simulink model "derivative_test"  (R2022b)
settings: Solver=FixedStepDiscrete  StartTime=0.0  StopTime=60  FixedStep=0.001  RelTol=1e-3
libraries: eeGeneralControl x2
settings Model: Creator=doann  LastModifiedBy=doann
settings OptimizationCC: DefaultParameterBehavior=Inlined  UseDivisionForNetSlopeComputation=on  GainParamInheritBuiltInType=on  UseFloatMulNetSlope=on  InlineInvariantSignals=on  PassReuseOutputArgsAs=Individual arguments  ZeroExternalMemoryAtStartup=off  ZeroInternalMemoryAtStartup=off  NoFixptDivByZeroProtection=on  EfficientFloat2IntCast=on  LifeSpan=1  OptimizeBlockOrder=speed  DifferentSizesBufferReuse=on  EfficientTunableParamExpr=on
settings DebuggingCC: ParameterTunabilityLossMsg=error
settings HardwareCC: ProdBitPerPointer=32  ProdBitPerSizeT=32  ProdBitPerPtrDiffT=32  ProdLargestAtomicInteger=Long  ProdLargestAtomicFloat=Double  ProdWordSize=32  ProdLongLongMode=on  ProdHWDeviceType=ARM Compatible->ARM Cortex-M
settings SFSimCC: MATLABDynamicMemAlloc=off
settings RTWCC: Description=Embedded Coder  SystemTargetFile=ert.tlc  GenCodeOnly=on  TemplateMakefile=ert_default_tmf  TargetLang=C++
settings CodeAppCC: ForceParamTrailComments=on  IgnoreCustomStorageClasses=off  OperatorAnnotations=on  SimulinkDataObjDesc=on  SFDataObjDesc=on  CustomSymbolStrGlobalVar=rt$N$M  CustomSymbolStrType=$N$M  CustomSymbolStrFcn=$N$M$F  CustomSymbolStrMacro=$N$M  InsertBlockDesc=on
settings ERTTargetCC: TargetLangStandard=C++11 (ISO)  GenerateSampleERTMain=on  IncludeMdlTerminateFcn=off  CombineSignalStateStructs=on  SuppressErrorStatus=on  SupportAbsoluteTime=off  CodeInterfacePackaging=C++ class  SupportComplex=off  InlinedParameterPlacement=NonHierarchical  RootIOFormat=Structure reference  ERTCustomFileTemplate=example_file_process.tlc  ERTFilePackagingFormat=CompactWithDataFile

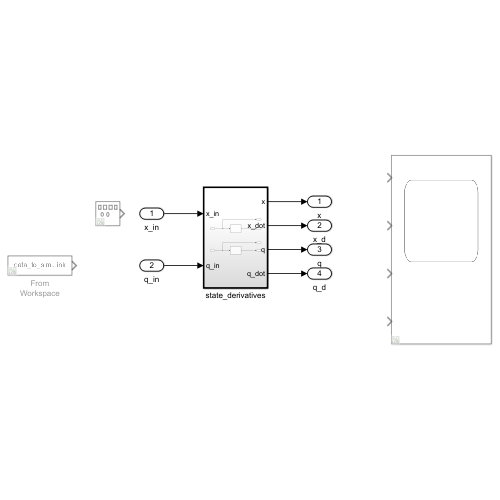
[thumbnail: Simulink's stored preview of the top-level diagram]
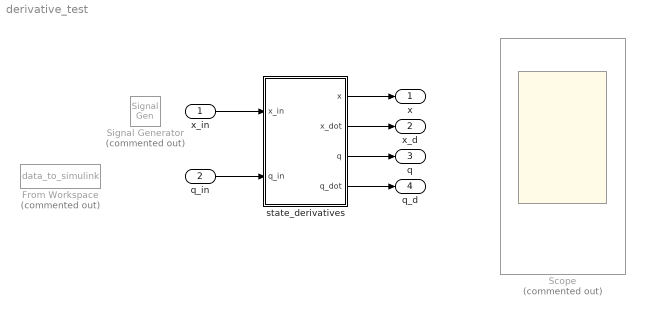
== system derivative_test ==
  x_in : Inport
  q_in : Inport  Port=2
  From Workspace : FromWorkspace  Commented=on  VariableName=data_to_simulink  SampleTime=0.001  OutputAfterFinalValue=Holding final value
  Scope : Scope  Commented=on  NumInputPorts=4
  Signal Generator : SignalGenerator  Commented=on  Amplitude=0.9  Frequency=pi  Units=rad/sec
  state_derivatives : Subsystem  TreatAsAtomicUnit=on  SystemSampleTime=0.001
  x : Outport
  x_d : Outport  Port=2
  q : Outport  Port=3
  q_d : Outport  Port=4
  wires:
  x_in/1 -> state_derivatives/1(x_in)
  q_in/1 -> state_derivatives/2(q_in)
  state_derivatives/1(x) -> x/1
  state_derivatives/2(x_dot) -> x_d/1
  state_derivatives/3(q) -> q/1
  state_derivatives/4(q_dot) -> q_d/1

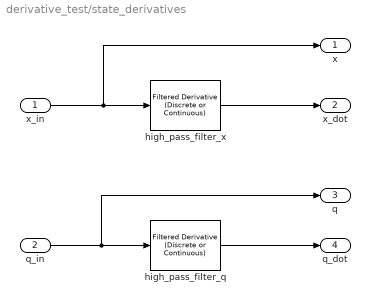
== system derivative_test/state_derivatives ==
  x_in : Inport
  q_in : Inport  Port=2
  high_pass_filter_q : eeGeneralControl/Filtered Derivative (Discrete or Continuous)  K=1  T=0.02  B=inf  A=-inf  minRatio=10  init_option=Inherited from block input  x0=0  Ts=0.001
      settings: LibrarySourceBlock=|
      | ee_sl_lib/General Control/Filtered Derivative
      | (Discrete or Continuous)
  high_pass_filter_x : eeGeneralControl/Filtered Derivative (Discrete or Continuous)  K=1  T=0.02  B=inf  A=-inf  minRatio=10  init_option=Inherited from block input  x0=0  Ts=0.001
      settings: LibrarySourceBlock=|
      | ee_sl_lib/General Control/Filtered Derivative
      | (Discrete or Continuous)
  x : Outport
  x_dot : Outport  Port=2
  q : Outport  Port=3
  q_dot : Outport  Port=4
  wires:
  x_in/1 -> x/1, high_pass_filter_x/1
  high_pass_filter_x/1 -> x_dot/1
  high_pass_filter_q/1 -> q_dot/1
  q_in/1 -> q/1, high_pass_filter_q/1
